simulink model "lab64"  (Simulink 8.0)
settings: Solver=ode45  StartTime=0.0  StopTime=inf  RelTol=1e-3
undefined symbols (not defined in the file): get, pskmod
libraries: commsink2 x3, commdigbbndpm3 x2, commeq2 x1, commchan3 x1, commrandsrc2 x1
settings Model: Creator=Dimav  LastModifiedBy=Dimav

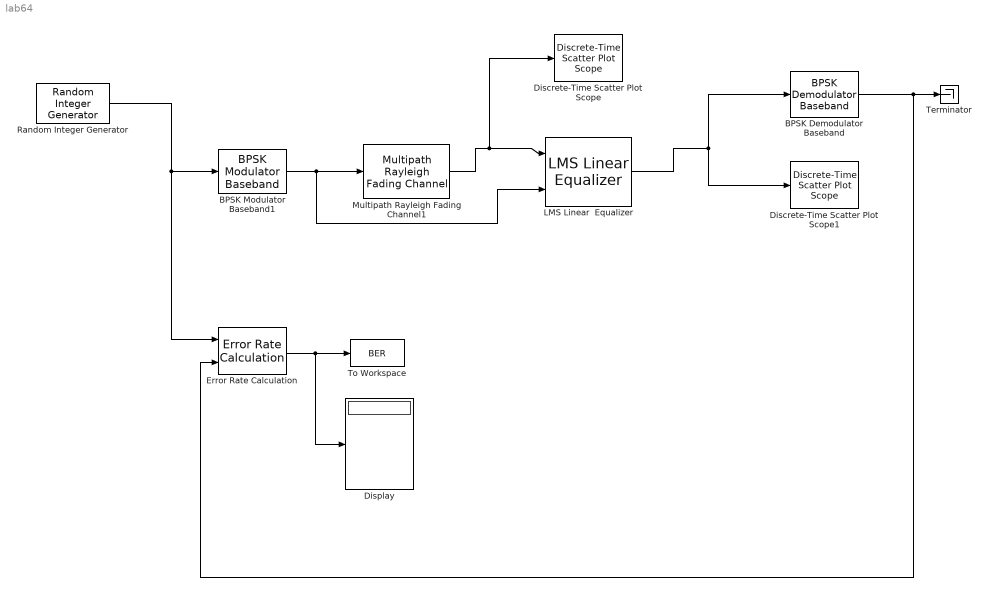
== system lab64 ==
  BPSK Demodulator Baseband : commdigbbndpm3/BPSK Demodulator Baseband  Ph=0  DecType=Hard decision  VarSource=Dialog  Variance=1  outDtype=boolean  derotateFactorWordLen=16
  BPSK Modulator Baseband1 : commdigbbndpm3/BPSK Modulator Baseband  Ph=0  outDtype=double  outWordLen=16  outUDDataType=sfix(16)  outFracLenMode=Best precision  outFracLen=15
  Discrete-Time Scatter Plot Scope : commsink2/Discrete-Time Scatter Plot Scope  Tag=ScatterPlot  sampPerSymb=1  offsetEye=0  numTraces=40  numNewFrames=40  LineMarkers=.  LineColors=b  fading=on  render=on  AxisGrid=on  xMin=-3.3  xMax=3.315  yMin=-3.3  yMax=3.315  inphaseLabel=In-phase Amplitude  quadratureLabel=Quadrature Amplitude  openScopeAtSimStart=on  FrameNumber=off  FigPos=get(0,'defaultfigureposition');  figTitle=Scatter Plot  numLinesMax=8  block_type_=scatter
  Discrete-Time Scatter Plot Scope1 : commsink2/Discrete-Time Scatter Plot Scope  Tag=ScatterPlot  sampPerSymb=1  offsetEye=0  numTraces=40  numNewFrames=40  LineMarkers=.  LineColors=b  fading=on  render=on  AxisGrid=on  xMin=-3.3  xMax=3.315  yMin=-3.3  yMax=3.315  inphaseLabel=In-phase Amplitude  quadratureLabel=Quadrature Amplitude  openScopeAtSimStart=on  FrameNumber=off  FigPos=get(0,'defaultfigureposition');  figTitle=Scatter Plot  numLinesMax=8  block_type_=scatter
  Display : Display
  Error Rate Calculation : commsink2/Error Rate Calculation  N=0  st_delay=0  cp_mode=Entire frame  subframe=[]  PMode=Port  WsName=ErrorVec  RsMode2=off  stop=on  numErr=200  maxBits=500
  LMS Linear  Equalizer : commeq2/LMS Linear  Equalizer  nTaps=4  nSamp=1  sigConst=pskmod([0:1],2);  delay=2  stepSize=0.1  leakage=1  initWeights=0  mode=off  outErr=off  outWeights=off
  Multipath Rayleigh Fading Channel1 : commchan3/Multipath Rayleigh Fading Channel  maxDopplerShift=100  spectrumType=Jakes  sigmaGaussian=1/sqrt(2)  coeffRounded=[1 -1.72 0.785]  freqMinMaxRJakes=[0 1]  freqMinMaxAJakes=[0 1]  sigmaGaussian1=1/sqrt(2)  sigmaGaussian2=1/sqrt(2)  centerFreqGaussian1=0.0  centerFreqGaussian2=0.0  gainGaussian1=0.5  gainGaussian2=0.5  coeffBell=9  dopplerSpectrum=doppler.jakes  pathDelays=1.0e-004 * [0 0.0400 0.0800 0.1200]  avgPathGaindB=[0 -3 -6 -9]  normalizePathGains=on  seed=73  enableProbe=1  openVisAtStart=on  outPathGains=off  outDelay=off
  Random Integer Generator : commrandsrc2/Random Integer Generator  mul=2  seed=37  Ts=1/500000  frameBased=on  sampPerFrame=8  orient=off  outDataType=boolean
  Terminator : Terminator
  To Workspace : ToWorkspace  VariableName=BER  SampleTime=-1  SaveFormat=Timeseries
  wires:
  Random Integer Generator/1 -> Error Rate Calculation/1, BPSK Modulator Baseband1/1
  Error Rate Calculation/1 -> To Workspace/1, Display/1
  BPSK Modulator Baseband1/1 -> LMS Linear  Equalizer/2, Multipath Rayleigh Fading Channel1/1
  Multipath Rayleigh Fading Channel1/1 -> Discrete-Time Scatter Plot Scope/1, LMS Linear  Equalizer/1
  BPSK Demodulator Baseband/1 -> Error Rate Calculation/2, Terminator/1
  LMS Linear  Equalizer/1 -> Discrete-Time Scatter Plot Scope1/1, BPSK Demodulator Baseband/1
